simulink model "Week2_problem1"  (R2020b)
settings: Solver=VariableStepAuto  StartTime=0.0  StopTime=10  RelTol=1e-3
settings Model: Creator=sai  LastModifiedBy=sai

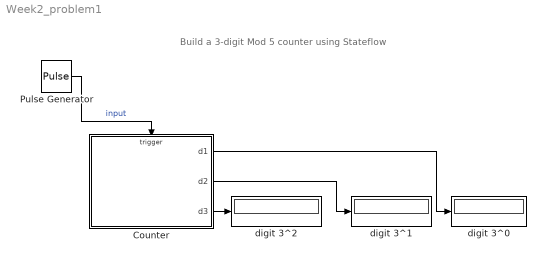
== system Week2_problem1 ==
  note: Build a 3-digit Mod 5 counter using Stateflow
  Counter : Stateflow chart  TreatAsAtomicUnit=on
  Pulse Generator : DiscretePulseGenerator  PulseType=Time based  Period=10  PulseWidth=5
  digit 3^0 : Display
  digit 3^1 : Display
  digit 3^2 : Display
  wires:
  Counter/1(d1) -> digit 3^0/1
  Pulse Generator/1 -> Counter/Trigger  "input"
  Counter/2(d2) -> digit 3^1/1
  Counter/3(d3) -> digit 3^2/1

== stateflow chart Week2_problem1/Counter ==
  settings: executeAtInitialization=1
  state digit1 [parallel]
    settings: executionOrder=1
    state Step1
      en: d1 = 1;
    state Step3
      en:
      d1=3;
    state Step2
      en:
      d1=2;
    state Step0
      en: d1 = 0;
    state Step4
      en: d1 = 4;
    digit1.Step2 -> digit1.Step3 : inputClick
    digit1.Step1 -> digit1.Step2 : inputClick
    digit1.Step0 -> digit1.Step1 : inputClick
    digit1.Step3 -> digit1.Step4
    (default) -> digit1.Step0
    digit1.Step4 -> digit1.Step0 : inputClick /{digit2.inc2;}
  state digit2 [parallel]
    settings: executionOrder=2
    state Step1
      en: d2 = 1;
    state Step3
      en: d2 = 3;
    state Step2
      en: d2 = 2;
    state Step4
      en: d2 = 4;
    state Step0
      en: d2 = 0;
    digit2.Step0 -> digit2.Step1 : inc2
    digit2.Step1 -> digit2.Step2 : inc2
    digit2.Step2 -> digit2.Step3 : inc2
    digit2.Step3 -> digit2.Step4 : inc2
    (default) -> digit2.Step0
    digit2.Step4 -> digit2.Step0 : inc2 /{digit3.inc3;}
  state digit3 [parallel]
    settings: executionOrder=3
    state Step1
      en: d3 = 1;
    state Step3
      en: d2 = 3;
    state Step2
      en: d2 = 2;
    state Step0
      en: d3 = 0;
    state Step4
      en: d3 = 4;
    digit3.Step0 -> digit3.Step1 : inc3
    digit3.Step2 -> digit3.Step3 : inc3
    digit3.Step1 -> digit3.Step2 : inc3
    digit3.Step3 -> digit3.Step4 : inc3
    (default) -> digit3.Step0
    digit3.Step4 -> digit3.Step0 : inc3
  data: d1 output size=1; d2 output size=1; d3 output size=1
  events: inc2 local EITHER_EDGE_EVENT; inc3 local EITHER_EDGE_EVENT; inputClick input EITHER_EDGE_EVENT
